simulink model "RS_O_yalmip"  (R2016b)
settings: Solver=ode1  StartTime=0.0  StopTime=T  FixedStep=1e-4  MaxStep=1e-3  RelTol=1e-6  EnableMultiTasking=on
InitFcn:
  | RS_O_script;
values from neighbouring files (symbols this model uses):
  C1 = 1e-9    (= 1e-09)    [Dati_MPC.m]
  C2 = 1e-9    (= 1e-09)    [Dati_MPC.m]
  Cext_Bp1 = Ce_Bp1*np_Bp1/ns_Bp1    (= 35750)    [Dati_MPC.m]
  Cext_Bp2 = Ce_Bp2*np_Bp2/ns_Bp2    (= 35750)    [Dati_MPC.m]
  Cext_BpM = Ce_BpM*np_BpM/ns_BpM    (= 68250)    [Dati_MPC.m]
  Cin_Bp1 = Ci_Bp1*np_Bp1/ns_Bp1    (= 16500)    [Dati_MPC.m]
  Cin_Bp2 = Ci_Bp2*np_Bp2/ns_Bp2    (= 16500)    [Dati_MPC.m]
  Cin_BpM = Ci_BpM*np_BpM/ns_BpM    (= 31500)    [Dati_MPC.m]
  Cint = 18e-3    (= 0.018)    [Dati_MPC.m]
  f = 50    [Dati_rete.m]
  ft_F = 10    [Dati_MPC.m]
  I_u = 0.1    [Dati_MPC.m]
  ki_PLL = w_t/Vd*(-w_t+sqrt(2*w_t^2-Vd^2*kp_PLL^2))    [Dati_MPC.m]
  kp_PLL = 0.9*kp_PLL_max    [Dati_MPC.m]
  MPCpar = struct    [Dati_MPC.m]    (also in Initialization.m)
  netdata = struct    [Dati_rete.m]
  P1 = 750e3    (= 750000)    [RS_O_script.m]
  P1v = 500e3    (= 500000)    [RS_O_script.m]
  P2 = 750e3    (= 750000)    [RS_O_script.m]
  P2v = 250e3    (= 250000)    [RS_O_script.m]
  P_u = 0.005    [Dati_MPC.m]
  Ppv1 = 500e3    (= 500000)    [Dati_MPC.m]
  Ppv2 = 850e3    (= 850000)    [Dati_MPC.m]
  Q1 = 350e3    (= 350000)    [RS_O_script.m]
  Q1v = 250e3    (= 250000)    [RS_O_script.m]
  Q2 = 300e3    (= 300000)    [RS_O_script.m]
  Q2v = 250e3    (= 250000)    [RS_O_script.m]
  Qbat1 = 50e3    (= 50000)    [Dati_MPC.m]
  Qbat2 = 50e3    (= 50000)    [Dati_MPC.m]
  Rext_Bp1 = Re_Bp1*ns_Bp1/np_Bp1    (= 0.0154545454545)    [Dati_MPC.m]
  Rext_Bp2 = Re_Bp2*ns_Bp2/np_Bp2    (= 0.0154545454545)    [Dati_MPC.m]
  Rext_BpM = Re_BpM*ns_BpM/np_BpM    (= 0.00809523809524)    [Dati_MPC.m]
  Rin_Bp1 = Ri_Bp1*ns_Bp1/np_Bp1    (= 0.363636363636)    [Dati_MPC.m]
  Rin_Bp2 = Ri_Bp2*ns_Bp2/np_Bp2    (= 0.363636363636)    [Dati_MPC.m]
  Rin_BpM = Ri_BpM*ns_BpM/np_BpM    (= 0.190476190476)    [Dati_MPC.m]
  SOC_10 = (Vbat1-Vbat1_min)/(Vbat1_max-Vbat1_min)    (= 0.625)    [Dati_MPC.m]
  SOC_20 = (Vbat2-Vbat2_min)/(Vbat2_max-Vbat2_min)    (= 0.625)    [Dati_MPC.m]
  SOC_M0 = (VbatM-VbatM_min)/(VbatM_max-VbatM_min)    (= 0.625)    [Dati_MPC.m]
  Srif = 1e6    (= 1000000)    [Dati_rete.m]
  t1 = 50    [RS_O_script.m]
  t2 = 110    [RS_O_script.m]
  t3 = 170    [RS_O_script.m]
  t_start_MPC = 10    [RS_O_script.m]
  tPLL = 2    [RS_O_script.m]
  Vbat1_max = 1.2*Vbat1_min    (= 480)    [Dati_MPC.m]
  Vbat1_min = 400    [Dati_MPC.m]
  Vbat2_max = 1.2*Vbat2_min    (= 480)    [Dati_MPC.m]
  Vbat2_min = 400    [Dati_MPC.m]
  VbatM_max = 1.2*VbatM_min    (= 480)    [Dati_MPC.m]
  VbatM_min = 400    [Dati_MPC.m]
  Vdc_1 = 800    [Dati_MPC.m]
  Vdc_2 = 800    [Dati_MPC.m]
  Vdc_M = 800    [Dati_MPC.m]
  Vrif_M = sqrt(2)/sqrt(3)*20e3    [Dati_MPC.m]
  Zrif = Vrif^2/Srif    (= 400)    [Dati_rete.m]
undefined symbols (not defined in the file or in its folder): Cfsc, Csc, j, L2, Lf, magnitude, Rc, Rint, Rsc
libraries: powerlib x87, powerlib_meascontrol x58, simulink x2
(part 2 of 3)

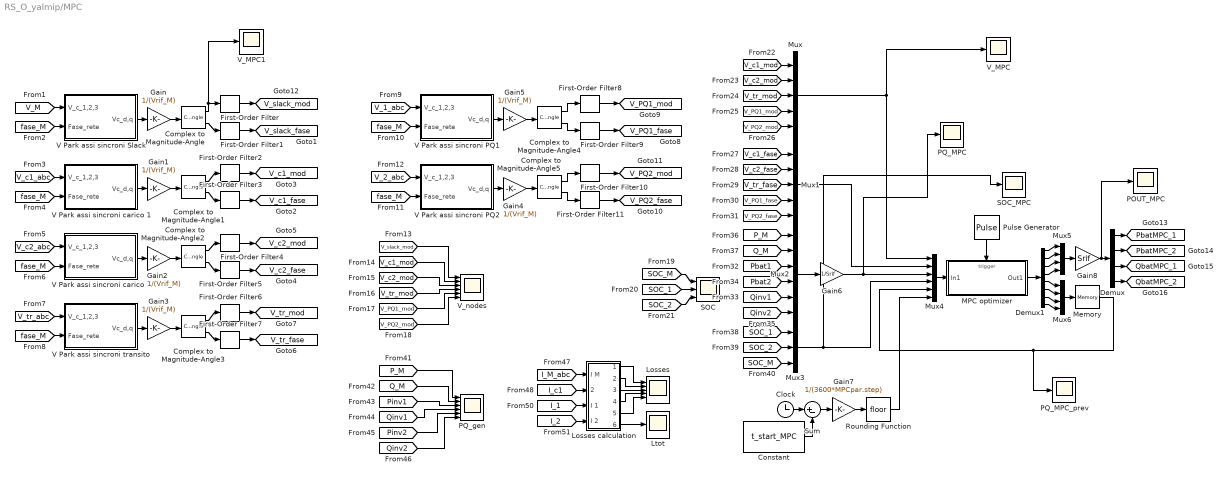
== system RS_O_yalmip/MPC ==
  Clock : Clock
  Complex to Magnitude-Angle{,1..5} (6 alike) : ComplexToMagnitudeAngle
  Constant : Constant  Value=t_start_MPC
  Demux : Demux
  Demux1 : Demux  Outputs=8
  First-Order Filter{,1..11} (12 alike) : powerlib_meascontrol/Filters/First-Order Filter  FilterType=Lowpass  Tc=1/(2*pi*ft_F)  Ts=0  Initialize=on  Vac_Init=[0, 0, 60]  Vdc_Init=0  PlotResponse=off  FreqRange="[0,  200,  1]"
  Gain{,1..5} (6 alike) : Gain  Gain=1/(Vrif_M)
  Gain6 : Gain  Gain=1/Srif
  Gain7 : Gain  Gain=1/(3600*MPCpar.step)
  Gain8 : Gain  Gain=Srif
  Losses : Scope  NumInputPorts=5
  Losses calculation : Subsystem
  Ltot : Scope
  MPC optimizer : Subsystem  TreatAsAtomicUnit=on
  Memory : Memory
  Mux : Mux  Inputs=5
  Mux1 : Mux  Inputs=5
  Mux2 : Mux  Inputs=6
  Mux3 : Mux  Inputs=3
  Mux4 : Mux  Inputs=6
  Mux5 : Mux
  Mux6 : Mux
  POUT_MPC : Scope
  PQ_MPC : Scope
  PQ_MPC_prev : Scope
  PQ_gen : Scope  NumInputPorts=6
  Pulse Generator : DiscretePulseGenerator  PulseType=Time based  Period=MPCpar.step*3600  PulseWidth=5  PhaseDelay=t_start_MPC
  Rounding Function : Rounding
  SOC : Scope  NumInputPorts=3
  SOC_MPC : Scope
  Sum : Sum  Inputs=|+-
  V Park assi sincroni PQ1 : Subsystem
  V Park assi sincroni PQ2 : Subsystem
  V Park assi sincroni Slack : Subsystem
  V Park assi sincroni carico 1 : Subsystem
  V Park assi sincroni carico 2 : Subsystem
  V Park assi sincroni transito : Subsystem
  V_MPC : Scope
  V_MPC1 : Scope
  V_nodes : Scope  NumInputPorts=6
  tag scope: PbatMPC_1=global, PbatMPC_2=global, QbatMPC_1=global, QbatMPC_2=global, V_PQ1_fase=global, V_PQ1_mod=global, V_PQ2_fase=global, V_PQ2_mod=global, V_c1_fase=global, V_c1_mod=global, V_c2_fase=global, V_c2_mod=global, V_slack_fase=global, V_slack_mod=global, V_tr_fase=global, V_tr_mod=global
  wires:
  [fase_M] -> V Park assi sincroni Slack/2(Fase_rete)
  [V_M] -> V Park assi sincroni Slack/1(V_c_1,2,3)
  [fase_M] -> V Park assi sincroni carico 1/2(Fase_rete)
  [V_c1_abc] -> V Park assi sincroni carico 1/1(V_c_1,2,3)
  [fase_M] -> V Park assi sincroni carico 2/2(Fase_rete)
  [V_c2_abc] -> V Park assi sincroni carico 2/1(V_c_1,2,3)
  [fase_M] -> V Park assi sincroni transito/2(Fase_rete)
  [V_tr_abc] -> V Park assi sincroni transito/1(V_c_1,2,3)
  [fase_M] -> V Park assi sincroni PQ1/2(Fase_rete)
  [V_1_abc] -> V Park assi sincroni PQ1/1(V_c_1,2,3)
  [fase_M] -> V Park assi sincroni PQ2/2(Fase_rete)
  [V_2_abc] -> V Park assi sincroni PQ2/1(V_c_1,2,3)
  V Park assi sincroni Slack/1(Vc_d,q) -> Gain/1
  Complex to Magnitude-Angle/1 -> V_MPC1/1, First-Order Filter/1
  Complex to Magnitude-Angle/2 -> First-Order Filter1/1
  Complex to Magnitude-Angle1/1 -> First-Order Filter2/1
  Complex to Magnitude-Angle1/2 -> First-Order Filter3/1
  V Park assi sincroni carico 1/1(Vc_d,q) -> Gain1/1
  Complex to Magnitude-Angle2/1 -> First-Order Filter4/1
  Complex to Magnitude-Angle2/2 -> First-Order Filter5/1
  V Park assi sincroni carico 2/1(Vc_d,q) -> Gain2/1
  Complex to Magnitude-Angle3/1 -> First-Order Filter6/1
  Complex to Magnitude-Angle3/2 -> First-Order Filter7/1
  V Park assi sincroni transito/1(Vc_d,q) -> Gain3/1
  Complex to Magnitude-Angle4/1 -> First-Order Filter8/1
  Complex to Magnitude-Angle4/2 -> First-Order Filter9/1
  V Park assi sincroni PQ1/1(Vc_d,q) -> Gain5/1
  Complex to Magnitude-Angle5/1 -> First-Order Filter10/1
  Complex to Magnitude-Angle5/2 -> First-Order Filter11/1
  V Park assi sincroni PQ2/1(Vc_d,q) -> Gain4/1
  [V_slack_mod] -> V_nodes/1
  [V_c1_mod] -> V_nodes/2
  [V_c2_mod] -> V_nodes/3
  [V_tr_mod] -> V_nodes/4
  [V_PQ1_mod] -> V_nodes/5
  [V_PQ2_mod] -> V_nodes/6
  Gain/1 -> Complex to Magnitude-Angle/1
  Gain1/1 -> Complex to Magnitude-Angle1/1
  Gain2/1 -> Complex to Magnitude-Angle2/1
  Gain3/1 -> Complex to Magnitude-Angle3/1
  Gain5/1 -> Complex to Magnitude-Angle4/1
  Gain4/1 -> Complex to Magnitude-Angle5/1
  [SOC_M] -> SOC/1
  [SOC_1] -> SOC/2
  [SOC_2] -> SOC/3
  First-Order Filter/1 -> [V_slack_mod]
  First-Order Filter1/1 -> [V_slack_fase]
  First-Order Filter2/1 -> [V_c1_mod]
  First-Order Filter3/1 -> [V_c1_fase]
  First-Order Filter4/1 -> [V_c2_mod]
  First-Order Filter5/1 -> [V_c2_fase]
  First-Order Filter6/1 -> [V_tr_mod]
  First-Order Filter7/1 -> [V_tr_fase]
  First-Order Filter8/1 -> [V_PQ1_mod]
  First-Order Filter9/1 -> [V_PQ1_fase]
  First-Order Filter10/1 -> [V_PQ2_mod]
  First-Order Filter11/1 -> [V_PQ2_fase]
  [V_c1_mod] -> Mux/1
  [V_c2_mod] -> Mux/2
  [V_tr_mod] -> Mux/3
  [V_PQ1_mod] -> Mux/4
  [V_PQ2_mod] -> Mux/5
  [V_c1_fase] -> Mux1/1
  [V_c2_fase] -> Mux1/2
  [V_tr_fase] -> Mux1/3
  [V_PQ1_fase] -> Mux1/4
  [V_PQ2_fase] -> Mux1/5
  [Qinv2] -> Mux2/6
  [Qinv1] -> Mux2/5
  [Pbat2] -> Mux2/4
  [Pbat1] -> Mux2/3
  [P_M] -> Mux2/1
  [Q_M] -> Mux2/2
  [SOC_1] -> Mux3/1
  [SOC_2] -> Mux3/2
  [SOC_M] -> Mux3/3
  Mux/1 -> Mux4/1, V_MPC/1
  Mux1/1 -> Mux4/2
  Mux2/1 -> Gain6/1
  Gain6/1 -> PQ_MPC/1, Mux4/3
  Mux3/1 -> SOC_MPC/1, Mux4/4
  Mux4/1 -> MPC optimizer/1(In1)
  Pulse Generator/1 -> MPC optimizer/Trigger
  Demux/1 -> [PbatMPC_1]
  Demux/2 -> [PbatMPC_2]
  Demux/4 -> [QbatMPC_2]
  Demux/3 -> [QbatMPC_1]
  Clock/1 -> Sum/1
  Constant/1 -> Sum/2
  Sum/1 -> Gain7/1
  Gain7/1 -> Rounding Function/1
  MPC optimizer/1(Out1) -> Demux1/1
  Mux5/1 -> Gain8/1
  Demux1/1 -> Mux5/1
  Demux1/2 -> Mux5/2
  Demux1/3 -> Mux5/3
  Demux1/4 -> Mux5/4
  Demux1/5 -> Mux6/1
  Demux1/6 -> Mux6/2
  Demux1/7 -> Mux6/3
  Demux1/8 -> Mux6/4
  Mux6/1 -> Memory/1
  Rounding Function/1 -> Mux4/6
  Memory/1 -> PQ_MPC_prev/1, Mux4/5
  Gain8/1 -> POUT_MPC/1, Demux/1
  [P_M] -> PQ_gen/1
  [Q_M] -> PQ_gen/2
  [Pinv1] -> PQ_gen/3
  [Qinv1] -> PQ_gen/4
  [Pinv2] -> PQ_gen/5
  [Qinv2] -> PQ_gen/6
  [I_M_abc] -> Losses calculation/1(I M)
  [I_c1] -> Losses calculation/2(I C1)
  [I_1] -> Losses calculation/3(I 1)
  [I_2] -> Losses calculation/4(I 2)
  Losses calculation/1(L12) -> Losses/1
  Losses calculation/2(L23) -> Losses/2
  Losses calculation/3(L34) -> Losses/3
  Losses calculation/4(L45) -> Losses/4
  Losses calculation/5(L46) -> Losses/5
  Losses calculation/6(Ltot) -> Ltot/1

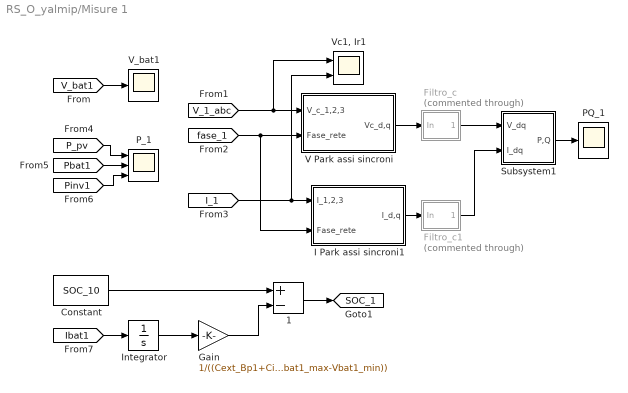
== system RS_O_yalmip/Misure 1 ==
  1 : Sum  Inputs=+-
  Constant : Constant  Value=SOC_10
  Filtro_c : Subsystem  Commented=through
  Filtro_c1 : Subsystem  Commented=through
  Gain : Gain  Gain=1/((Cext_Bp1+Cin_Bp1)*(Vbat1_max-Vbat1_min))
  I Park assi sincroni1 : Subsystem
  Integrator : Integrator
  PQ_1 : Scope
  P_1 : Scope  NumInputPorts=3
  Subsystem1 : Subsystem
  V Park assi sincroni : Subsystem
  V_bat1 : Scope
  "Vc1, Ir1" : Scope  NumInputPorts=2
  tag scope: SOC_1=global
  wires:
  I Park assi sincroni1/1(I_d,q) -> Filtro_c1/1(In)
  V Park assi sincroni/1(Vc_d,q) -> Filtro_c/1(In)
  [fase_1] -> V Park assi sincroni/2(Fase_rete), I Park assi sincroni1/2(Fase_rete)
  [I_1] -> "Vc1, Ir1"/2, I Park assi sincroni1/1(I_1,2,3)
  Subsystem1/1(P,Q) -> PQ_1/1
  [V_1_abc] -> V Park assi sincroni/1(V_c_1,2,3), "Vc1, Ir1"/1
  [P_pv] -> P_1/1
  [Pbat1] -> P_1/2
  [Pinv1] -> P_1/3
  [V_bat1] -> V_bat1/1
  [Ibat1] -> Integrator/1
  Integrator/1 -> Gain/1
  Constant/1 -> 1/1
  1/1 -> [SOC_1]
  Gain/1 -> 1/2
  Filtro_c/1(Out) -> Subsystem1/1(V_dq)
  Filtro_c1/1(Out) -> Subsystem1/2(I_dq)

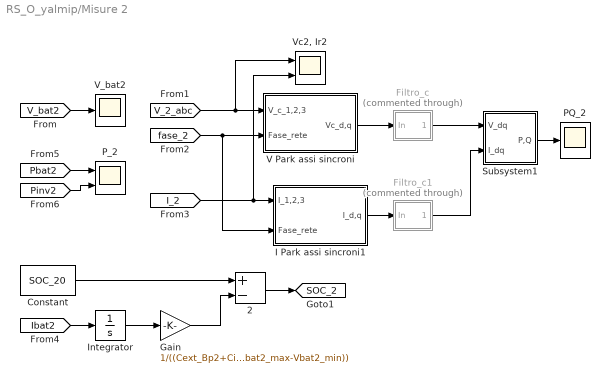
== system RS_O_yalmip/Misure 2 ==
  2 : Sum  Inputs=+-
  Constant : Constant  Value=SOC_20
  Filtro_c : Subsystem  Commented=through
  Filtro_c1 : Subsystem  Commented=through
  Gain : Gain  Gain=1/((Cext_Bp2+Cin_Bp2)*(Vbat2_max-Vbat2_min))
  I Park assi sincroni1 : Subsystem
  Integrator : Integrator
  PQ_2 : Scope
  P_2 : Scope  NumInputPorts=2
  Subsystem1 : Subsystem
  V Park assi sincroni : Subsystem
  V_bat2 : Scope
  "Vc2, Ir2" : Scope  NumInputPorts=2
  tag scope: SOC_2=global
  wires:
  [V_2_abc] -> "Vc2, Ir2"/1, V Park assi sincroni/1(V_c_1,2,3)
  Subsystem1/1(P,Q) -> PQ_2/1
  [I_2] -> I Park assi sincroni1/1(I_1,2,3), "Vc2, Ir2"/2
  [fase_2] -> I Park assi sincroni1/2(Fase_rete), V Park assi sincroni/2(Fase_rete)
  V Park assi sincroni/1(Vc_d,q) -> Filtro_c/1(In)
  I Park assi sincroni1/1(I_d,q) -> Filtro_c1/1(In)
  [V_bat2] -> V_bat2/1
  [Pinv2] -> P_2/2
  [Pbat2] -> P_2/1
  [Ibat2] -> Integrator/1
  Integrator/1 -> Gain/1
  Constant/1 -> 2/1
  2/1 -> [SOC_2]
  Gain/1 -> 2/2
  Filtro_c1/1(Out) -> Subsystem1/2(I_dq)
  Filtro_c/1(Out) -> Subsystem1/1(V_dq)

== system RS_O_yalmip/Misure Carichi ==
  First-Order Filter{,1..3} (4 alike) : powerlib_meascontrol/Filters/First-Order Filter  FilterType=Lowpass  Tc=1/(2*pi*ft_F)  Ts=0  Initialize=on  Vac_Init=[0, 0, 60]  Vdc_Init=0  PlotResponse=off  FreqRange="[0,  200,  1]"
  PQ_c1 : Scope  NumInputPorts=2
  PQ_c2 : Scope  NumInputPorts=2
  P_c1,2 : Scope  NumInputPorts=4
  "Power (3ph, Instantaneous)" : powerlib_meascontrol/Measurements/Power (3ph, Instantaneous)
  "Power (3ph, Instantaneous)1" : powerlib_meascontrol/Measurements/Power (3ph, Instantaneous)
  V,I_c1 : Scope  NumInputPorts=2
  V,I_c2 : Scope  NumInputPorts=2
  tag scope: Pc1=global, Pc2=global, Qc1=global, Qc2=global
  wires:
  [I_c1] -> "Power (3ph, Instantaneous)"/2, V,I_c1/2
  [V_c1_abc] -> "Power (3ph, Instantaneous)"/1, V,I_c1/1
  "Power (3ph, Instantaneous)"/2 -> First-Order Filter1/1
  "Power (3ph, Instantaneous)1"/2 -> First-Order Filter3/1
  "Power (3ph, Instantaneous)1"/1 -> First-Order Filter2/1
  [I_c2] -> "Power (3ph, Instantaneous)1"/2, V,I_c2/2
  [V_c2_abc] -> "Power (3ph, Instantaneous)1"/1, V,I_c2/1
  "Power (3ph, Instantaneous)"/1 -> First-Order Filter/1
  First-Order Filter/1 -> [Pc1], P_c1,2/1, PQ_c1/1
  First-Order Filter1/1 -> P_c1,2/2, [Qc1], PQ_c1/2
  First-Order Filter2/1 -> P_c1,2/3, [Pc2], PQ_c2/1
  First-Order Filter3/1 -> P_c1,2/4, [Qc2], PQ_c2/2

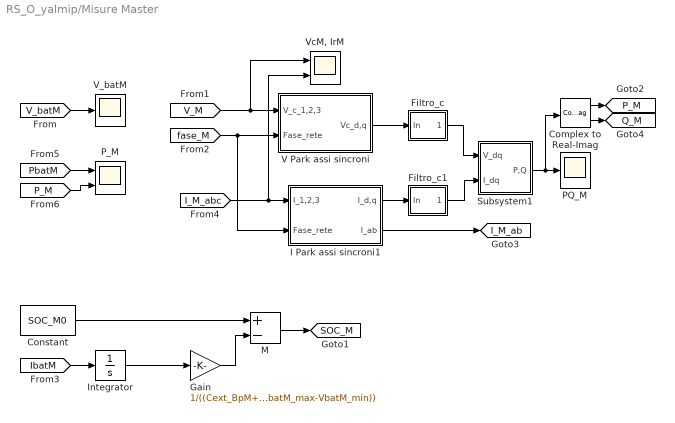
== system RS_O_yalmip/Misure Master ==
  Complex to Real-Imag : ComplexToRealImag
  Constant : Constant  Value=SOC_M0
  Filtro_c : Subsystem
  Filtro_c1 : Subsystem
  Gain : Gain  Gain=1/((Cext_BpM+Cin_BpM)*(VbatM_max-VbatM_min))
  I Park assi sincroni1 : Subsystem
  Integrator : Integrator
  M : Sum  Inputs=+-
  PQ_M : Scope
  P_M : Scope  NumInputPorts=2
  Subsystem1 : Subsystem
  V Park assi sincroni : Subsystem
  V_batM : Scope
  "VcM, IrM" : Scope  NumInputPorts=2
  tag scope: I_M_ab=global, P_M=global, Q_M=global, SOC_M=global
  wires:
  Subsystem1/1(P,Q) -> PQ_M/1, Complex to Real-Imag/1
  [I_M_abc] -> I Park assi sincroni1/1(I_1,2,3), "VcM, IrM"/2
  [fase_M] -> I Park assi sincroni1/2(Fase_rete), V Park assi sincroni/2(Fase_rete)
  [V_M] -> "VcM, IrM"/1, V Park assi sincroni/1(V_c_1,2,3)
  I Park assi sincroni1/2(I_ab) -> [I_M_ab]
  V Park assi sincroni/1(Vc_d,q) -> Filtro_c/1(In)
  I Park assi sincroni1/1(I_d,q) -> Filtro_c1/1(In)
  [P_M] -> P_M/2
  [PbatM] -> P_M/1
  [V_batM] -> V_batM/1
  [IbatM] -> Integrator/1
  Integrator/1 -> Gain/1
  Constant/1 -> M/1
  M/1 -> [SOC_M]
  Gain/1 -> M/2
  Filtro_c/1(Out) -> Subsystem1/1(V_dq)
  Filtro_c1/1(Out) -> Subsystem1/2(I_dq)
  Complex to Real-Imag/2 -> [Q_M]
  Complex to Real-Imag/1 -> [P_M]

== system RS_O_yalmip/Misure transito ==
  Subsystem2 : Subsystem
  Three-Phase Series RLC Load2 : powerlib/Elements/Three-Phase Series RLC Load  LConnTagsString=A|B|C  Configuration=Y (floating)  NominalVoltage=20e3  Vabc=[1e3 1e3 1e3]  Vabcp=[1e3 1e3 1e3]  NominalFrequency=50  UnbalancedPower=off  ActivePower=0.1  InductivePower=0  CapacitivePower=0  Pabc=[10e3 9e3 11e3]  QLabc=[100 90 110]  QCabc=[100 90 110]  Pabcp=[10e3 9e3 11e3]  QLabcp=[100 90 110]  QCabcp=[100 90 110]  Measurements=None  LoadType=constant PQ
  Three-Phase V-I Measurement2 : powerlib/Measurements/Three-Phase V-I Measurement  VoltageMeasurement=phase-to-phase  SetLabelV=off  LabelV=Vabc  Vpu=off  VpuLL=off  CurrentMeasurement=no  SetLabelI=off  LabelI=Iabc  Ipu=off  Pbase=100e6  Vbase=500e3  OutputType=Complex  PhasorSimulation=off  PSBequivalent=0
  A : PMIOPort  Port=1  Side=Left
  B : PMIOPort  Port=2  Side=Left
  C : PMIOPort  Port=3  Side=Left
  tag scope: V_tr_abc=global
  wires:
  Three-Phase V-I Measurement2/1 -> Subsystem2/1(V_c)
  Subsystem2/1(V_f) -> [V_tr_abc]
  connections:
  Three-Phase V-I Measurement2/RConn1 -- Three-Phase Series RLC Load2/LConn1
  Three-Phase Series RLC Load2/LConn3 -- Three-Phase V-I Measurement2/RConn3
  Three-Phase Series RLC Load2/LConn2 -- Three-Phase V-I Measurement2/RConn2
  Three-Phase V-I Measurement2/LConn2 -- B/RConn1
  Three-Phase V-I Measurement2/LConn3 -- C/RConn1
  Three-Phase V-I Measurement2/LConn1 -- A/RConn1

== system RS_O_yalmip/Carico1/PLL ==
  V_a,b : Inport
  Add1 : Sum
  Complex to Real-Imag : ComplexToRealImag  Output=Imag
  Complex to Real-Imag1 : ComplexToRealImag  Output=Real
  Constant2 : Constant  Value=50
  Filtro_c : Subsystem
  Gain2 : Gain  Gain=-j
  Gain3 : Gain  Gain=2*pi
  Integrator : Integrator  WrapState=on
  Math Function1 : Math  SaturateOnIntegerOverflow=on
  PI_fase : Subsystem
  Product1 : Product
  Vs : Outport
  Fase : Outport  Port=2
  wires:
  Complex to Real-Imag1/1 -> Vs/1
  Add1/1 -> Integrator/1
  Filtro_c/1(Out) -> Complex to Real-Imag1/1
  V_a,b/1 -> Product1/1
  Integrator/1 -> Gain2/1, Fase/1
  Complex to Real-Imag/1 -> PI_fase/1(dI)
  Product1/1 -> Complex to Real-Imag/1, Filtro_c/1(In)
  Constant2/1 -> Gain3/1
  Gain3/1 -> Add1/2
  Gain2/1 -> Math Function1/1
  Math Function1/1 -> Product1/2
  PI_fase/1(dw) -> Add1/1

== system RS_O_yalmip/Carico1/Park su assi fissi ==
  V_1,2,3 : Inport
  Add : Sum  Inputs=+++
  Constant : Constant  Value=exp(j*2*pi/3)
  Constant1 : Constant  Value=exp(j*4*pi/3)
  Demux : Demux  Outputs=3
  Gain : Gain  Gain=2/3
  Product : Product
  Product1 : Product
  V_s : Outport
  wires:
  Demux/2 -> Product/1
  Product/1 -> Add/2
  Product1/1 -> Add/3
  Constant/1 -> Product/2
  Constant1/1 -> Product1/2
  Add/1 -> Gain/1
  Demux/3 -> Product1/1
  Gain/1 -> V_s/1
  V_1,2,3/1 -> Demux/1
  Demux/1 -> Add/1

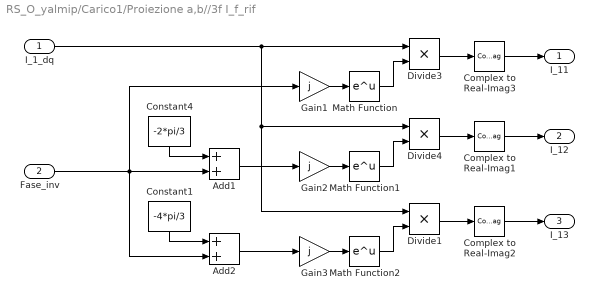
== system RS_O_yalmip/Carico1/Proiezione a,b//3f I_f_rif ==
  I_1_dq : Inport
  Fase_inv : Inport  Port=2
  Add1 : Sum
  Add2 : Sum
  Complex to Real-Imag1 : ComplexToRealImag  Output=Real
  Complex to Real-Imag2 : ComplexToRealImag  Output=Real
  Complex to Real-Imag3 : ComplexToRealImag  Output=Real
  Constant1 : Constant  Value=-4*pi/3
  Constant4 : Constant  Value=-2*pi/3
  Divide1 : Product  Inputs=**
  Divide3 : Product  Inputs=**
  Divide4 : Product  Inputs=**
  Gain1 : Gain  Gain=j
  Gain2 : Gain  Gain=j
  Gain3 : Gain  Gain=j
  Math Function : Math  SaturateOnIntegerOverflow=on
  Math Function1 : Math  SaturateOnIntegerOverflow=on
  Math Function2 : Math  SaturateOnIntegerOverflow=on
  I_11 : Outport
  I_12 : Outport  Port=2
  I_13 : Outport  Port=3
  wires:
  Constant1/1 -> Add2/1
  Constant4/1 -> Add1/1
  Fase_inv/1 -> Add1/2, Add2/2, Gain1/1
  Add2/1 -> Gain3/1
  Add1/1 -> Gain2/1
  Math Function2/1 -> Divide1/2
  Gain3/1 -> Math Function2/1
  I_1_dq/1 -> Divide3/1, Divide4/1, Divide1/1
  Math Function1/1 -> Divide4/2
  Gain2/1 -> Math Function1/1
  Math Function/1 -> Divide3/2
  Gain1/1 -> Math Function/1
  Complex to Real-Imag2/1 -> I_13/1
  Complex to Real-Imag1/1 -> I_12/1
  Complex to Real-Imag3/1 -> I_11/1
  Divide1/1 -> Complex to Real-Imag2/1
  Divide4/1 -> Complex to Real-Imag1/1
  Divide3/1 -> Complex to Real-Imag3/1

== system RS_O_yalmip/Carico1/Ritardo_PLL1 ==
  P : Inport
  Divide6 : Product  Inputs=**
  Step : Step  Time=tPLL  SampleTime=0
  g : Outport
  wires:
  P/1 -> Divide6/1
  Divide6/1 -> g/1
  Step/1 -> Divide6/2

== system RS_O_yalmip/Carico1/Ritardo_PLL2 ==
  P : Inport
  Divide6 : Product  Inputs=**
  Step : Step  Time=tPLL  SampleTime=0
  g : Outport
  wires:
  Step/1 -> Divide6/2
  Divide6/1 -> g/1
  P/1 -> Divide6/1

== system RS_O_yalmip/Carico1/Ritardo_PLL7 ==
  P : Inport
  Divide6 : Product  Inputs=**
  Step : Step  Time=tPLL  SampleTime=0
  g : Outport
  wires:
  Step/1 -> Divide6/2
  Divide6/1 -> g/1
  P/1 -> Divide6/1

== system RS_O_yalmip/Carico1/Subsystem ==
  P : Inport
  Q : Inport  Port=2
  V : Inport  Port=3
  Divide5 : Product  Inputs=*/
  Divide6 : Product  Inputs=*/
  First-Order Filter : powerlib_meascontrol/Filters/First-Order Filter  FilterType=Lowpass  Tc=1/(2*pi*ft_F)  Ts=0  Initialize=on  Vac_Init=[0, 0, 60]  Vdc_Init=0  PlotResponse=off  FreqRange="[0,  200,  1]"
  First-Order Filter1 : powerlib_meascontrol/Filters/First-Order Filter  FilterType=Lowpass  Tc=1/(2*pi*ft_F)  Ts=0  Initialize=on  Vac_Init=[0, 0, 60]  Vdc_Init=0  PlotResponse=off  FreqRange="[0,  200,  1]"
  Gain : Gain  Gain=2/3
  Gain2 : Gain  Gain=2/3
  Gain3 : Gain  Gain=-1
  Real-Imag to Complex : RealImagToComplex
  Saturation : Saturate  UpperLimit=inf  LowerLimit=1e-6
  I_dq : Outport
  wires:
  Gain3/1 -> Divide6/2
  V/1 -> Saturation/1
  Real-Imag to Complex/1 -> I_dq/1
  P/1 -> Gain/1
  Gain2/1 -> Divide6/1
  Gain/1 -> Divide5/1
  Q/1 -> Gain2/1
  Saturation/1 -> Divide5/2, Gain3/1
  Divide5/1 -> First-Order Filter/1
  Divide6/1 -> First-Order Filter1/1
  First-Order Filter/1 -> Real-Imag to Complex/1
  First-Order Filter1/1 -> Real-Imag to Complex/2

== system RS_O_yalmip/Carico1/Subsystem1 ==
  V_c : Inport
  Add : Sum  Inputs=+-
  Add1 : Sum  Inputs=+-
  Add2 : Sum  Inputs=+-
  Demux : Demux  Outputs=3
  Gain : Gain  Gain=1/3
  Gain1 : Gain  Gain=1/3
  Gain2 : Gain  Gain=1/3
  Mux2 : Mux  Inputs=3
  V_f : Outport
  wires:
  Mux2/1 -> V_f/1
  Demux/1 -> Gain/1
  Gain/1 -> Add1/2, Add/1
  Demux/2 -> Gain1/1
  Gain2/1 -> Add/2, Add2/1
  Gain1/1 -> Add2/2, Add1/1
  Add/1 -> Mux2/1
  Add1/1 -> Mux2/2
  Add2/1 -> Mux2/3
  V_c/1 -> Demux/1
  Demux/3 -> Gain2/1

== system RS_O_yalmip/Carico2/PLL ==
  V_a,b : Inport
  Add1 : Sum
  Complex to Real-Imag : ComplexToRealImag  Output=Imag
  Complex to Real-Imag1 : ComplexToRealImag  Output=Real
  Constant2 : Constant  Value=50
  Filtro_c : Subsystem
  Gain2 : Gain  Gain=-j
  Gain3 : Gain  Gain=2*pi
  Integrator : Integrator  WrapState=on
  Math Function1 : Math  SaturateOnIntegerOverflow=on
  PI_fase : Subsystem
  Product1 : Product
  Vs : Outport
  Fase : Outport  Port=2
  wires:
  Complex to Real-Imag1/1 -> Vs/1
  Add1/1 -> Integrator/1
  Filtro_c/1(Out) -> Complex to Real-Imag1/1
  V_a,b/1 -> Product1/1
  Integrator/1 -> Gain2/1, Fase/1
  Complex to Real-Imag/1 -> PI_fase/1(dI)
  Product1/1 -> Complex to Real-Imag/1, Filtro_c/1(In)
  Constant2/1 -> Gain3/1
  Gain3/1 -> Add1/2
  Gain2/1 -> Math Function1/1
  Math Function1/1 -> Product1/2
  PI_fase/1(dw) -> Add1/1

== system RS_O_yalmip/Carico2/Park su assi fissi ==
  V_1,2,3 : Inport
  Add : Sum  Inputs=+++
  Constant : Constant  Value=exp(j*2*pi/3)
  Constant1 : Constant  Value=exp(j*4*pi/3)
  Demux : Demux  Outputs=3
  Gain : Gain  Gain=2/3
  Product : Product
  Product1 : Product
  V_s : Outport
  wires:
  Demux/2 -> Product/1
  Product/1 -> Add/2
  Product1/1 -> Add/3
  Constant/1 -> Product/2
  Constant1/1 -> Product1/2
  Add/1 -> Gain/1
  Demux/3 -> Product1/1
  Gain/1 -> V_s/1
  V_1,2,3/1 -> Demux/1
  Demux/1 -> Add/1

== system RS_O_yalmip/Carico2/Proiezione a,b//3f I_f_rif ==
  I_1_dq : Inport
  Fase_inv : Inport  Port=2
  Add1 : Sum
  Add2 : Sum
  Complex to Real-Imag1 : ComplexToRealImag  Output=Real
  Complex to Real-Imag2 : ComplexToRealImag  Output=Real
  Complex to Real-Imag3 : ComplexToRealImag  Output=Real
  Constant1 : Constant  Value=-4*pi/3
  Constant4 : Constant  Value=-2*pi/3
  Divide1 : Product  Inputs=**
  Divide3 : Product  Inputs=**
  Divide4 : Product  Inputs=**
  Gain1 : Gain  Gain=j
  Gain2 : Gain  Gain=j
  Gain3 : Gain  Gain=j
  Math Function : Math  SaturateOnIntegerOverflow=on
  Math Function1 : Math  SaturateOnIntegerOverflow=on
  Math Function2 : Math  SaturateOnIntegerOverflow=on
  I_11 : Outport
  I_12 : Outport  Port=2
  I_13 : Outport  Port=3
  wires:
  Constant1/1 -> Add2/1
  Constant4/1 -> Add1/1
  Fase_inv/1 -> Add1/2, Add2/2, Gain1/1
  Add2/1 -> Gain3/1
  Add1/1 -> Gain2/1
  Math Function2/1 -> Divide1/2
  Gain3/1 -> Math Function2/1
  I_1_dq/1 -> Divide3/1, Divide4/1, Divide1/1
  Math Function1/1 -> Divide4/2
  Gain2/1 -> Math Function1/1
  Math Function/1 -> Divide3/2
  Gain1/1 -> Math Function/1
  Complex to Real-Imag2/1 -> I_13/1
  Complex to Real-Imag1/1 -> I_12/1
  Complex to Real-Imag3/1 -> I_11/1
  Divide1/1 -> Complex to Real-Imag2/1
  Divide4/1 -> Complex to Real-Imag1/1
  Divide3/1 -> Complex to Real-Imag3/1

== system RS_O_yalmip/Carico2/Ritardo_PLL1 ==
  P : Inport
  Divide6 : Product  Inputs=**
  Step : Step  Time=tPLL  SampleTime=0
  g : Outport
  wires:
  P/1 -> Divide6/1
  Divide6/1 -> g/1
  Step/1 -> Divide6/2

== system RS_O_yalmip/Carico2/Ritardo_PLL2 ==
  P : Inport
  Divide6 : Product  Inputs=**
  Step : Step  Time=tPLL  SampleTime=0
  g : Outport
  wires:
  Step/1 -> Divide6/2
  Divide6/1 -> g/1
  P/1 -> Divide6/1

== system RS_O_yalmip/Carico2/Ritardo_PLL7 ==
  P : Inport
  Divide6 : Product  Inputs=**
  Step : Step  Time=tPLL  SampleTime=0
  g : Outport
  wires:
  Step/1 -> Divide6/2
  Divide6/1 -> g/1
  P/1 -> Divide6/1

== system RS_O_yalmip/Carico2/Subsystem ==
  P : Inport
  Q : Inport  Port=2
  V : Inport  Port=3
  Divide5 : Product  Inputs=*/
  Divide6 : Product  Inputs=*/
  First-Order Filter : powerlib_meascontrol/Filters/First-Order Filter  FilterType=Lowpass  Tc=1/(2*pi*ft_F)  Ts=0  Initialize=on  Vac_Init=[0, 0, 60]  Vdc_Init=0  PlotResponse=off  FreqRange="[0,  200,  1]"
  First-Order Filter1 : powerlib_meascontrol/Filters/First-Order Filter  FilterType=Lowpass  Tc=1/(2*pi*ft_F)  Ts=0  Initialize=on  Vac_Init=[0, 0, 60]  Vdc_Init=0  PlotResponse=off  FreqRange="[0,  200,  1]"
  Gain : Gain  Gain=2/3
  Gain2 : Gain  Gain=2/3
  Gain3 : Gain  Gain=-1
  Real-Imag to Complex : RealImagToComplex
  Saturation : Saturate  UpperLimit=inf  LowerLimit=1e-6
  I_dq : Outport
  wires:
  Gain3/1 -> Divide6/2
  V/1 -> Saturation/1
  Real-Imag to Complex/1 -> I_dq/1
  P/1 -> Gain/1
  Gain2/1 -> Divide6/1
  Gain/1 -> Divide5/1
  Q/1 -> Gain2/1
  Saturation/1 -> Divide5/2, Gain3/1
  Divide5/1 -> First-Order Filter/1
  Divide6/1 -> First-Order Filter1/1
  First-Order Filter/1 -> Real-Imag to Complex/1
  First-Order Filter1/1 -> Real-Imag to Complex/2

== system RS_O_yalmip/Carico2/Subsystem1 ==
  V_c : Inport
  Add : Sum  Inputs=+-
  Add1 : Sum  Inputs=+-
  Add2 : Sum  Inputs=+-
  Demux : Demux  Outputs=3
  Gain : Gain  Gain=1/3
  Gain1 : Gain  Gain=1/3
  Gain2 : Gain  Gain=1/3
  Mux2 : Mux  Inputs=3
  V_f : Outport
  wires:
  Mux2/1 -> V_f/1
  Demux/1 -> Gain/1
  Gain/1 -> Add1/2, Add/1
  Demux/2 -> Gain1/1
  Gain2/1 -> Add/2, Add2/1
  Gain1/1 -> Add2/2, Add1/1
  Add/1 -> Mux2/1
  Add1/1 -> Mux2/2
  Add2/1 -> Mux2/3
  V_c/1 -> Demux/1
  Demux/3 -> Gain2/1

== system RS_O_yalmip/Controllo 1/PLL ==
  V_a,b : Inport
  Add1 : Sum
  Complex to Real-Imag : ComplexToRealImag  Output=Imag
  Complex to Real-Imag1 : ComplexToRealImag  Output=Real
  Constant2 : Constant  Value=50
  Filtro_c : Subsystem
  Gain2 : Gain  Gain=-j
  Gain3 : Gain  Gain=2*pi
  Integrator : Integrator  WrapState=on
  Math Function1 : Math  SaturateOnIntegerOverflow=on
  PI_fase : Subsystem
  Product1 : Product
  Vs : Outport
  Fase : Outport  Port=2
  wires:
  Complex to Real-Imag1/1 -> Vs/1
  Add1/1 -> Integrator/1
  Filtro_c/1(Out) -> Complex to Real-Imag1/1
  V_a,b/1 -> Product1/1
  Integrator/1 -> Gain2/1, Fase/1
  Complex to Real-Imag/1 -> PI_fase/1(dI)
  Product1/1 -> Complex to Real-Imag/1, Filtro_c/1(In)
  Constant2/1 -> Gain3/1
  Gain3/1 -> Add1/2
  Gain2/1 -> Math Function1/1
  Math Function1/1 -> Product1/2
  PI_fase/1(dw) -> Add1/1

== system RS_O_yalmip/Controllo 1/Park su assi fissi ==
  V_1,2,3 : Inport
  Add : Sum  Inputs=+++
  Constant : Constant  Value=exp(j*2*pi/3)
  Constant1 : Constant  Value=exp(j*4*pi/3)
  Demux : Demux  Outputs=3
  Gain : Gain  Gain=2/3
  Product : Product
  Product1 : Product
  V_s : Outport
  wires:
  Demux/2 -> Product/1
  Product/1 -> Add/2
  Product1/1 -> Add/3
  Constant/1 -> Product/2
  Constant1/1 -> Product1/2
  Add/1 -> Gain/1
  Demux/3 -> Product1/1
  Gain/1 -> V_s/1
  V_1,2,3/1 -> Demux/1
  Demux/1 -> Add/1

== system RS_O_yalmip/Controllo 1/Proiezione a,b//3f I_f_rif ==
  I_1_dq : Inport
  Fase_inv : Inport  Port=2
  Add1 : Sum
  Add2 : Sum
  Complex to Real-Imag1 : ComplexToRealImag  Output=Real
  Complex to Real-Imag2 : ComplexToRealImag  Output=Real
  Complex to Real-Imag3 : ComplexToRealImag  Output=Real
  Constant1 : Constant  Value=-4*pi/3
  Constant4 : Constant  Value=-2*pi/3
  Divide1 : Product  Inputs=**
  Divide3 : Product  Inputs=**
  Divide4 : Product  Inputs=**
  Gain1 : Gain  Gain=j
  Gain2 : Gain  Gain=j
  Gain3 : Gain  Gain=j
  Math Function : Math  SaturateOnIntegerOverflow=on
  Math Function1 : Math  SaturateOnIntegerOverflow=on
  Math Function2 : Math  SaturateOnIntegerOverflow=on
  I_11 : Outport
  I_12 : Outport  Port=2
  I_13 : Outport  Port=3
  wires:
  Constant1/1 -> Add2/1
  Constant4/1 -> Add1/1
  Fase_inv/1 -> Add1/2, Add2/2, Gain1/1
  Add2/1 -> Gain3/1
  Add1/1 -> Gain2/1
  Math Function2/1 -> Divide1/2
  Gain3/1 -> Math Function2/1
  I_1_dq/1 -> Divide3/1, Divide4/1, Divide1/1
  Math Function1/1 -> Divide4/2
  Gain2/1 -> Math Function1/1
  Math Function/1 -> Divide3/2
  Gain1/1 -> Math Function/1
  Complex to Real-Imag2/1 -> I_13/1
  Complex to Real-Imag1/1 -> I_12/1
  Complex to Real-Imag3/1 -> I_11/1
  Divide1/1 -> Complex to Real-Imag2/1
  Divide4/1 -> Complex to Real-Imag1/1
  Divide3/1 -> Complex to Real-Imag3/1

== system RS_O_yalmip/Controllo 1/Ritardo_PLL1 ==
  P : Inport
  Divide6 : Product  Inputs=**
  Step : Step  Time=tPLL  SampleTime=0
  g : Outport
  wires:
  P/1 -> Divide6/1
  Divide6/1 -> g/1
  Step/1 -> Divide6/2

== system RS_O_yalmip/Controllo 1/Ritardo_PLL2 ==
  P : Inport
  Divide6 : Product  Inputs=**
  Step : Step  Time=tPLL  SampleTime=0
  g : Outport
  wires:
  Step/1 -> Divide6/2
  Divide6/1 -> g/1
  P/1 -> Divide6/1

== system RS_O_yalmip/Controllo 1/Ritardo_PLL3 ==
  P : Inport
  Divide6 : Product  Inputs=**
  Step : Step  Time=tPLL  SampleTime=0
  g : Outport
  wires:
  P/1 -> Divide6/1
  Divide6/1 -> g/1
  Step/1 -> Divide6/2

== system RS_O_yalmip/Controllo 1/Ritardo_PLL7 ==
  P : Inport
  Divide6 : Product  Inputs=**
  Step : Step  Time=tPLL  SampleTime=0
  g : Outport
  wires:
  Step/1 -> Divide6/2
  Divide6/1 -> g/1
  P/1 -> Divide6/1

== system RS_O_yalmip/Controllo 1/Subsystem ==
  P : Inport
  Q : Inport  Port=2
  V : Inport  Port=3
  Divide5 : Product  Inputs=*/
  Divide6 : Product  Inputs=*/
  First-Order Filter : powerlib_meascontrol/Filters/First-Order Filter  Commented=through  FilterType=Lowpass  Tc=1/(2*pi*ft_F)  Ts=0  Initialize=on  Vac_Init=[0, 0, 60]  Vdc_Init=0  PlotResponse=off  FreqRange="[0,  200,  1]"
  First-Order Filter1 : powerlib_meascontrol/Filters/First-Order Filter  Commented=through  FilterType=Lowpass  Tc=1/(2*pi*ft_F)  Ts=0  Initialize=on  Vac_Init=[0, 0, 60]  Vdc_Init=0  PlotResponse=off  FreqRange="[0,  200,  1]"
  Gain : Gain  Gain=2/3
  Gain2 : Gain  Gain=2/3
  Gain3 : Gain  Gain=-1
  Real-Imag to Complex : RealImagToComplex
  Saturation : Saturate  UpperLimit=inf  LowerLimit=1e-6
  I_dq : Outport
  wires:
  Gain3/1 -> Divide6/2
  V/1 -> Saturation/1
  Real-Imag to Complex/1 -> I_dq/1
  P/1 -> Gain/1
  Gain2/1 -> Divide6/1
  Gain/1 -> Divide5/1
  Q/1 -> Gain2/1
  Saturation/1 -> Divide5/2, Gain3/1
  Divide5/1 -> First-Order Filter/1
  Divide6/1 -> First-Order Filter1/1
  First-Order Filter/1 -> Real-Imag to Complex/1
  First-Order Filter1/1 -> Real-Imag to Complex/2

== system RS_O_yalmip/Controllo 2/PLL ==
  V_a,b : Inport
  Add1 : Sum
  Complex to Real-Imag : ComplexToRealImag  Output=Imag
  Complex to Real-Imag1 : ComplexToRealImag  Output=Real
  Constant2 : Constant  Value=50
  Filtro_c : Subsystem
  Gain2 : Gain  Gain=-j
  Gain3 : Gain  Gain=2*pi
  Integrator : Integrator  WrapState=on
  Math Function1 : Math  SaturateOnIntegerOverflow=on
  PI_fase : Subsystem
  Product1 : Product
  Vs : Outport
  Fase : Outport  Port=2
  wires:
  Complex to Real-Imag1/1 -> Vs/1
  Add1/1 -> Integrator/1
  Filtro_c/1(Out) -> Complex to Real-Imag1/1
  V_a,b/1 -> Product1/1
  Integrator/1 -> Gain2/1, Fase/1
  Complex to Real-Imag/1 -> PI_fase/1(dI)
  Product1/1 -> Complex to Real-Imag/1, Filtro_c/1(In)
  Constant2/1 -> Gain3/1
  Gain3/1 -> Add1/2
  Gain2/1 -> Math Function1/1
  Math Function1/1 -> Product1/2
  PI_fase/1(dw) -> Add1/1

== system RS_O_yalmip/Controllo 2/Park su assi fissi ==
  V_1,2,3 : Inport
  Add : Sum  Inputs=+++
  Constant : Constant  Value=exp(j*2*pi/3)
  Constant1 : Constant  Value=exp(j*4*pi/3)
  Demux : Demux  Outputs=3
  Gain : Gain  Gain=2/3
  Product : Product
  Product1 : Product
  V_s : Outport
  wires:
  Demux/2 -> Product/1
  Product/1 -> Add/2
  Product1/1 -> Add/3
  Constant/1 -> Product/2
  Constant1/1 -> Product1/2
  Add/1 -> Gain/1
  Demux/3 -> Product1/1
  Gain/1 -> V_s/1
  V_1,2,3/1 -> Demux/1
  Demux/1 -> Add/1

== system RS_O_yalmip/Controllo 2/Proiezione a,b//3f I_f_rif ==
  I_1_dq : Inport
  Fase_inv : Inport  Port=2
  Add1 : Sum
  Add2 : Sum
  Complex to Real-Imag1 : ComplexToRealImag  Output=Real
  Complex to Real-Imag2 : ComplexToRealImag  Output=Real
  Complex to Real-Imag3 : ComplexToRealImag  Output=Real
  Constant1 : Constant  Value=-4*pi/3
  Constant4 : Constant  Value=-2*pi/3
  Divide1 : Product  Inputs=**
  Divide3 : Product  Inputs=**
  Divide4 : Product  Inputs=**
  Gain1 : Gain  Gain=j
  Gain2 : Gain  Gain=j
  Gain3 : Gain  Gain=j
  Math Function : Math  SaturateOnIntegerOverflow=on
  Math Function1 : Math  SaturateOnIntegerOverflow=on
  Math Function2 : Math  SaturateOnIntegerOverflow=on
  I_11 : Outport
  I_12 : Outport  Port=2
  I_13 : Outport  Port=3
  wires:
  Constant1/1 -> Add2/1
  Constant4/1 -> Add1/1
  Fase_inv/1 -> Add1/2, Add2/2, Gain1/1
  Add2/1 -> Gain3/1
  Add1/1 -> Gain2/1
  Math Function2/1 -> Divide1/2
  Gain3/1 -> Math Function2/1
  I_1_dq/1 -> Divide3/1, Divide4/1, Divide1/1
  Math Function1/1 -> Divide4/2
  Gain2/1 -> Math Function1/1
  Math Function/1 -> Divide3/2
  Gain1/1 -> Math Function/1
  Complex to Real-Imag2/1 -> I_13/1
  Complex to Real-Imag1/1 -> I_12/1
  Complex to Real-Imag3/1 -> I_11/1
  Divide1/1 -> Complex to Real-Imag2/1
  Divide4/1 -> Complex to Real-Imag1/1
  Divide3/1 -> Complex to Real-Imag3/1

== system RS_O_yalmip/Controllo 2/Ritardo_PLL1 ==
  P : Inport
  Divide6 : Product  Inputs=**
  Step : Step  Time=tPLL  SampleTime=0
  g : Outport
  wires:
  P/1 -> Divide6/1
  Divide6/1 -> g/1
  Step/1 -> Divide6/2

== system RS_O_yalmip/Controllo 2/Ritardo_PLL2 ==
  P : Inport
  Divide6 : Product  Inputs=**
  Step : Step  Time=tPLL  SampleTime=0
  g : Outport
  wires:
  Step/1 -> Divide6/2
  Divide6/1 -> g/1
  P/1 -> Divide6/1

== system RS_O_yalmip/Controllo 2/Ritardo_PLL3 ==
  P : Inport
  Divide6 : Product  Inputs=**
  Step : Step  Time=tPLL  SampleTime=0
  g : Outport
  wires:
  P/1 -> Divide6/1
  Divide6/1 -> g/1
  Step/1 -> Divide6/2

== system RS_O_yalmip/Controllo 2/Ritardo_PLL7 ==
  P : Inport
  Divide6 : Product  Inputs=**
  Step : Step  Time=tPLL  SampleTime=0
  g : Outport
  wires:
  Step/1 -> Divide6/2
  Divide6/1 -> g/1
  P/1 -> Divide6/1

== system RS_O_yalmip/Controllo 2/Subsystem ==
  P : Inport
  Q : Inport  Port=2
  V : Inport  Port=3
  Divide5 : Product  Inputs=*/
  Divide6 : Product  Inputs=*/
  First-Order Filter : powerlib_meascontrol/Filters/First-Order Filter  Commented=through  FilterType=Lowpass  Tc=1/(2*pi*ft_F)  Ts=0  Initialize=on  Vac_Init=[0, 0, 60]  Vdc_Init=0  PlotResponse=off  FreqRange="[0,  200,  1]"
  First-Order Filter1 : powerlib_meascontrol/Filters/First-Order Filter  Commented=through  FilterType=Lowpass  Tc=1/(2*pi*ft_F)  Ts=0  Initialize=on  Vac_Init=[0, 0, 60]  Vdc_Init=0  PlotResponse=off  FreqRange="[0,  200,  1]"
  Gain : Gain  Gain=2/3
  Gain2 : Gain  Gain=2/3
  Gain3 : Gain  Gain=-1
  Real-Imag to Complex : RealImagToComplex
  Saturation : Saturate  UpperLimit=inf  LowerLimit=1e-6
  I_dq : Outport
  wires:
  Gain3/1 -> Divide6/2
  V/1 -> Saturation/1
  Real-Imag to Complex/1 -> I_dq/1
  P/1 -> Gain/1
  Gain2/1 -> Divide6/1
  Gain/1 -> Divide5/1
  Q/1 -> Gain2/1
  Saturation/1 -> Divide5/2, Gain3/1
  Divide5/1 -> First-Order Filter/1
  Divide6/1 -> First-Order Filter1/1
  First-Order Filter/1 -> Real-Imag to Complex/1
  First-Order Filter1/1 -> Real-Imag to Complex/2

== system RS_O_yalmip/Controllo Master/Media complessa ==
  w : Inport
  fase : Inport  Port=2
  I_a,b : Inport  Port=3
  Complex to Real-Imag : ComplexToRealImag
  Divide3 : Product  Inputs=**
  Filtro_c1 : Subsystem
  Gain : Gain  Gain=1/(2*pi)
  Gain1 : Gain  Gain=-j
  Math Function : Math  SaturateOnIntegerOverflow=on
  Mean (Variable Frequency) : powerlib_meascontrol/Measurements/Mean (Variable Frequency)  Finit=50  Fmin=45  Vinit=0  Ts=0
  Mean (Variable Frequency)1 : powerlib_meascontrol/Measurements/Mean (Variable Frequency)  Finit=50  Fmin=45  Vinit=0  Ts=0
  Real-Imag to Complex : RealImagToComplex
  I_dc_d,q : Outport
  wires:
  I_a,b/1 -> Complex to Real-Imag/1
  Complex to Real-Imag/1 -> Mean (Variable Frequency)/2
  Complex to Real-Imag/2 -> Mean (Variable Frequency)1/2
  Mean (Variable Frequency)/1 -> Real-Imag to Complex/1
  Mean (Variable Frequency)1/1 -> Real-Imag to Complex/2
  w/1 -> Gain/1
  Gain/1 -> Mean (Variable Frequency)1/1, Mean (Variable Frequency)/1
  Gain1/1 -> Math Function/1
  Math Function/1 -> Divide3/2
  Divide3/1 -> I_dc_d,q/1
  fase/1 -> Gain1/1
  Real-Imag to Complex/1 -> Filtro_c1/1(In)
  Filtro_c1/1(Out) -> Divide3/1

== system RS_O_yalmip/Controllo Master/PI Complesso ==
  In1 : Inport
  Complex to Real-Imag : ComplexToRealImag
  Gain1 : Gain  Gain=-1
  PID Controller : simulink/Continuous/PID Controller  Controller=PI  TimeDomain=Continuous-time  SampleTime=-1  IntegratorMethod=Forward Euler  FilterMethod=Forward Euler  Form=Parallel  UseFilter=on  ControllerParametersSource=internal  P=P_u  I=I_u  D=0  N=100  InitialConditionSource=internal  InitialConditionForIntegrator=0  InitialConditionForFilter=0  ExternalReset=none  LimitOutput=off  UpperSaturationLimit=inf  LowerSaturationLimit=-inf  LinearizeAsGain=on  AntiWindupMode=none  Kb=1  TrackingMode=off  Kt=1  PParamMin=[]  PParamMax=[]  IParamMin=[]  IParamMax=[]  DParamMin=[]  DParamMax=[]  NParamMin=[]  NParamMax=[]  KbParamMin=[]  KbParamMax=[]  KtParamMin=[]  KtParamMax=[]  POutMin=[]  POutMax=[]  IOutMin=[]  IOutMax=[]  DOutMin=[]  DOutMax=[]  NOutMin=[]  NOutMax=[]  KbOutMin=[]  KbOutMax=[]  KtOutMin=[]  KtOutMax=[]  IntegratorOutMin=[]  IntegratorOutMax=[]  FilterOutMin=[]  FilterOutMax=[]  SumOutMin=[]  SumOutMax=[]  SumI1OutMin=[]  SumI1OutMax=[]  SumI2OutMin=[]  SumI2OutMax=[]  SumI3OutMin=[]  SumI3OutMax=[]  SumDOutMin=[]  SumDOutMax=[]  SaturationOutMin=[]  SaturationOutMax=[]  IntegratorContinuousStateAttributes=''  IntegratorStateMustResolveToSignalObject=off  IntegratorRTWStateStorageClass=Auto  FilterContinuousStateAttributes=''  FilterStateMustResolveToSignalObject=off  FilterRTWStateStorageClass=Auto  DifferentiatorICPrevScaledInput=0  DifferentiatorOutMin=[]  DifferentiatorOutMax=[]
  PID Controller1 : simulink/Continuous/PID Controller  Controller=PI  TimeDomain=Continuous-time  SampleTime=-1  IntegratorMethod=Forward Euler  FilterMethod=Forward Euler  Form=Parallel  UseFilter=on  ControllerParametersSource=internal  P=P_u  I=I_u  D=0  N=100  InitialConditionSource=internal  InitialConditionForIntegrator=0  InitialConditionForFilter=0  ExternalReset=none  LimitOutput=off  UpperSaturationLimit=inf  LowerSaturationLimit=-inf  LinearizeAsGain=on  AntiWindupMode=none  Kb=1  TrackingMode=off  Kt=1  PParamMin=[]  PParamMax=[]  IParamMin=[]  IParamMax=[]  DParamMin=[]  DParamMax=[]  NParamMin=[]  NParamMax=[]  KbParamMin=[]  KbParamMax=[]  KtParamMin=[]  KtParamMax=[]  POutMin=[]  POutMax=[]  IOutMin=[]  IOutMax=[]  DOutMin=[]  DOutMax=[]  NOutMin=[]  NOutMax=[]  KbOutMin=[]  KbOutMax=[]  KtOutMin=[]  KtOutMax=[]  IntegratorOutMin=[]  IntegratorOutMax=[]  FilterOutMin=[]  FilterOutMax=[]  SumOutMin=[]  SumOutMax=[]  SumI1OutMin=[]  SumI1OutMax=[]  SumI2OutMin=[]  SumI2OutMax=[]  SumI3OutMin=[]  SumI3OutMax=[]  SumDOutMin=[]  SumDOutMax=[]  SaturationOutMin=[]  SaturationOutMax=[]  IntegratorContinuousStateAttributes=''  IntegratorStateMustResolveToSignalObject=off  IntegratorRTWStateStorageClass=Auto  FilterContinuousStateAttributes=''  FilterStateMustResolveToSignalObject=off  FilterRTWStateStorageClass=Auto  DifferentiatorICPrevScaledInput=0  DifferentiatorOutMin=[]  DifferentiatorOutMax=[]
  Real-Imag to Complex : RealImagToComplex
  Out1 : Outport
  wires:
  In1/1 -> Gain1/1
  Gain1/1 -> Complex to Real-Imag/1
  Complex to Real-Imag/1 -> PID Controller/1
  Complex to Real-Imag/2 -> PID Controller1/1
  PID Controller/1 -> Real-Imag to Complex/1
  PID Controller1/1 -> Real-Imag to Complex/2
  Real-Imag to Complex/1 -> Out1/1

== system RS_O_yalmip/Controllo Master/Proiezione a,b//3f I_f_rif ==
  V_M_dq : Inport
  Fase_inv : Inport  Port=2
  Add1 : Sum
  Add2 : Sum
  Complex to Real-Imag1 : ComplexToRealImag  Output=Real
  Complex to Real-Imag2 : ComplexToRealImag  Output=Real
  Complex to Real-Imag3 : ComplexToRealImag  Output=Real
  Constant1 : Constant  Value=-4*pi/3
  Constant4 : Constant  Value=-2*pi/3
  Divide1 : Product  Inputs=**
  Divide3 : Product  Inputs=**
  Divide4 : Product  Inputs=**
  Gain1 : Gain  Gain=j
  Gain2 : Gain  Gain=j
  Gain3 : Gain  Gain=j
  Math Function : Math  SaturateOnIntegerOverflow=on
  Math Function1 : Math  SaturateOnIntegerOverflow=on
  Math Function2 : Math  SaturateOnIntegerOverflow=on
  V_M1 : Outport
  V_M2 : Outport  Port=2
  V_M3 : Outport  Port=3
  wires:
  Divide3/1 -> Complex to Real-Imag3/1
  Divide4/1 -> Complex to Real-Imag1/1
  Divide1/1 -> Complex to Real-Imag2/1
  Complex to Real-Imag3/1 -> V_M1/1
  Complex to Real-Imag1/1 -> V_M2/1
  Complex to Real-Imag2/1 -> V_M3/1
  Gain1/1 -> Math Function/1
  Math Function/1 -> Divide3/2
  Gain2/1 -> Math Function1/1
  Math Function1/1 -> Divide4/2
  V_M_dq/1 -> Divide1/1, Divide4/1, Divide3/1
  Gain3/1 -> Math Function2/1
  Math Function2/1 -> Divide1/2
  Add1/1 -> Gain2/1
  Add2/1 -> Gain3/1
  Fase_inv/1 -> Gain1/1, Add2/2, Add1/2
  Constant4/1 -> Add1/1
  Constant1/1 -> Add2/1

== system RS_O_yalmip/DC PV/Ritardo_PLL2 ==
  P : Inport
  Divide6 : Product  Inputs=**
  Step : Step  Time=tPLL  SampleTime=0
  g : Outport
  wires:
  Step/1 -> Divide6/2
  Divide6/1 -> g/1
  P/1 -> Divide6/1

== system RS_O_yalmip/Inverter ID 1/Subsystem2 ==
  V_c : Inport
  Add : Sum  Inputs=+-
  Add1 : Sum  Inputs=+-
  Add2 : Sum  Inputs=+-
  Demux : Demux  Outputs=3
  Gain : Gain  Gain=1/3
  Gain1 : Gain  Gain=1/3
  Gain2 : Gain  Gain=1/3
  Mux2 : Mux  Inputs=3
  V_f : Outport
  wires:
  Mux2/1 -> V_f/1
  Demux/1 -> Gain/1
  Gain/1 -> Add1/2, Add/1
  Demux/2 -> Gain1/1
  Gain2/1 -> Add/2, Add2/1
  Gain1/1 -> Add2/2, Add1/1
  Add/1 -> Mux2/1
  Add1/1 -> Mux2/2
  Add2/1 -> Mux2/3
  V_c/1 -> Demux/1
  Demux/3 -> Gain2/1

== system RS_O_yalmip/Inverter ID 2/Subsystem2 ==
  V_c : Inport
  Add : Sum  Inputs=+-
  Add1 : Sum  Inputs=+-
  Add2 : Sum  Inputs=+-
  Demux : Demux  Outputs=3
  Gain : Gain  Gain=1/3
  Gain1 : Gain  Gain=1/3
  Gain2 : Gain  Gain=1/3
  Mux2 : Mux  Inputs=3
  V_f : Outport
  wires:
  Demux/3 -> Gain2/1
  V_c/1 -> Demux/1
  Add2/1 -> Mux2/3
  Add1/1 -> Mux2/2
  Add/1 -> Mux2/1
  Gain1/1 -> Add1/1, Add2/2
  Gain2/1 -> Add2/1, Add/2
  Demux/2 -> Gain1/1
  Gain/1 -> Add/1, Add1/2
  Demux/1 -> Gain/1
  Mux2/1 -> V_f/1

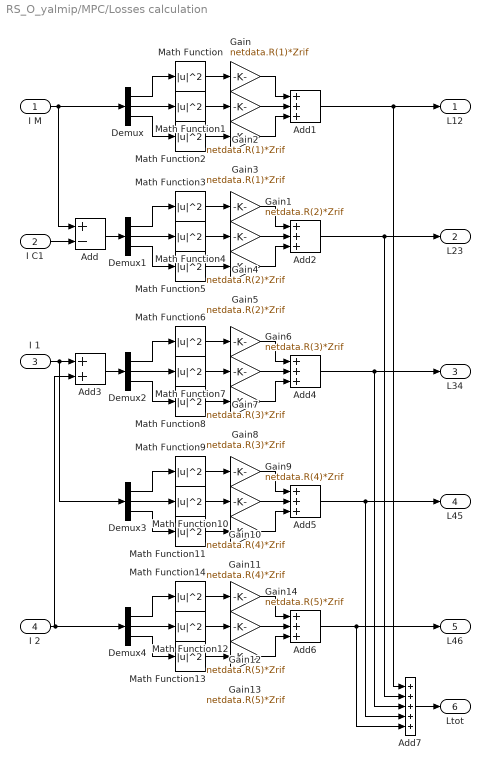
== system RS_O_yalmip/MPC/Losses calculation ==
  I M : Inport
  I C1 : Inport  Port=2
  I 1 : Inport  Port=3
  I 2 : Inport  Port=4
  Add : Sum  Inputs=+-
  Add{1..2,4..6} (5 alike) : Sum  Inputs=+++
  Add3 : Sum
  Add7 : Sum  Inputs=+++++
  Demux{,1..4} (5 alike) : Demux  Outputs=3
  Gain : Gain  Gain=netdata.R(1)*Zrif
  Gain1 : Gain  Gain=netdata.R(2)*Zrif
  Gain10 : Gain  Gain=netdata.R(4)*Zrif
  Gain11 : Gain  Gain=netdata.R(4)*Zrif
  Gain12 : Gain  Gain=netdata.R(5)*Zrif
  Gain13 : Gain  Gain=netdata.R(5)*Zrif
  Gain14 : Gain  Gain=netdata.R(5)*Zrif
  Gain2 : Gain  Gain=netdata.R(1)*Zrif
  Gain3 : Gain  Gain=netdata.R(1)*Zrif
  Gain4 : Gain  Gain=netdata.R(2)*Zrif
  Gain5 : Gain  Gain=netdata.R(2)*Zrif
  Gain6 : Gain  Gain=netdata.R(3)*Zrif
  Gain7 : Gain  Gain=netdata.R(3)*Zrif
  Gain8 : Gain  Gain=netdata.R(3)*Zrif
  Gain9 : Gain  Gain=netdata.R(4)*Zrif
  Math Function{,1..14} (15 alike) : Math  Operator=magnitude^2  SaturateOnIntegerOverflow=on
  L12 : Outport
  L23 : Outport  Port=2
  L34 : Outport  Port=3
  L45 : Outport  Port=4
  L46 : Outport  Port=5
  Ltot : Outport  Port=6
  wires:
  Math Function/1 -> Gain/1
  I C1/1 -> Add/2
  I M/1 -> Add/1, Demux/1
  Demux/1 -> Math Function/1
  Math Function1/1 -> Gain2/1
  Demux/2 -> Math Function1/1
  Math Function2/1 -> Gain3/1
  Demux/3 -> Math Function2/1
  Gain/1 -> Add1/1
  Gain2/1 -> Add1/2
  Gain3/1 -> Add1/3
  Add1/1 -> Add7/1, L12/1
  Math Function3/1 -> Gain1/1
  Demux1/1 -> Math Function3/1
  Math Function4/1 -> Gain4/1
  Demux1/2 -> Math Function4/1
  Math Function5/1 -> Gain5/1
  Demux1/3 -> Math Function5/1
  Gain1/1 -> Add2/1
  Gain4/1 -> Add2/2
  Gain5/1 -> Add2/3
  Add/1 -> Demux1/1
  Add2/1 -> Add7/2, L23/1
  Math Function6/1 -> Gain6/1
  Demux2/1 -> Math Function6/1
  Math Function7/1 -> Gain7/1
  Demux2/2 -> Math Function7/1
  Math Function8/1 -> Gain8/1
  Demux2/3 -> Math Function8/1
  Gain6/1 -> Add4/1
  Gain7/1 -> Add4/2
  Gain8/1 -> Add4/3
  Add3/1 -> Demux2/1
  Add4/1 -> Add7/3, L34/1
  I 2/1 -> Add3/2, Demux4/1
  Math Function9/1 -> Gain9/1
  I 1/1 -> Demux3/1, Add3/1
  Demux3/1 -> Math Function9/1
  Math Function10/1 -> Gain10/1
  Demux3/2 -> Math Function10/1
  Math Function11/1 -> Gain11/1
  Demux3/3 -> Math Function11/1
  Gain9/1 -> Add5/1
  Gain10/1 -> Add5/2
  Gain11/1 -> Add5/3
  Add5/1 -> Add7/4, L45/1
  Math Function14/1 -> Gain14/1
  Demux4/1 -> Math Function14/1
  Math Function12/1 -> Gain12/1
  Demux4/2 -> Math Function12/1
  Math Function13/1 -> Gain13/1
  Demux4/3 -> Math Function13/1
  Gain14/1 -> Add6/1
  Gain12/1 -> Add6/2
  Gain13/1 -> Add6/3
  Add6/1 -> Add7/5, L46/1
  Add7/1 -> Ltot/1

== system RS_O_yalmip/MPC/MPC optimizer ==
  In1 : Inport
  Trigger : TriggerPort  VariantControl=Variant
  Interpreted MATLAB Function : MATLABFcn  MATLABFcn=MPC_opt  OutputDimensions=8
  Out1 : Outport
  wires:
  Interpreted MATLAB Function/1 -> Out1/1
  In1/1 -> Interpreted MATLAB Function/1

== system RS_O_yalmip/MPC/V Park assi sincroni PQ1 ==
  V_c_1,2,3 : Inport
  Fase_rete : Inport  Port=2
  Add : Sum  Inputs=+++
  Constant : Constant  Value=exp(j*2*pi/3)
  Constant1 : Constant  Value=exp(j*4*pi/3)
  Demux : Demux  Outputs=3
  Gain : Gain  Gain=2/3
  Gain1 : Gain  Gain=-j
  Math Function : Math  SaturateOnIntegerOverflow=on
  Product : Product
  Product1 : Product
  Product2 : Product
  Vc_d,q : Outport
  wires:
  Fase_rete/1 -> Gain1/1
  Product2/1 -> Vc_d,q/1
  Gain1/1 -> Math Function/1
  Math Function/1 -> Product2/2
  Product/1 -> Add/2
  Product1/1 -> Add/3
  Constant/1 -> Product/2
  Constant1/1 -> Product1/2
  Add/1 -> Gain/1
  V_c_1,2,3/1 -> Demux/1
  Demux/1 -> Add/1
  Demux/2 -> Product/1
  Demux/3 -> Product1/1
  Gain/1 -> Product2/1

== system RS_O_yalmip/MPC/V Park assi sincroni PQ2 ==
  V_c_1,2,3 : Inport
  Fase_rete : Inport  Port=2
  Add : Sum  Inputs=+++
  Constant : Constant  Value=exp(j*2*pi/3)
  Constant1 : Constant  Value=exp(j*4*pi/3)
  Demux : Demux  Outputs=3
  Gain : Gain  Gain=2/3
  Gain1 : Gain  Gain=-j
  Math Function : Math  SaturateOnIntegerOverflow=on
  Product : Product
  Product1 : Product
  Product2 : Product
  Vc_d,q : Outport
  wires:
  Gain/1 -> Product2/1
  Demux/3 -> Product1/1
  Demux/2 -> Product/1
  Demux/1 -> Add/1
  V_c_1,2,3/1 -> Demux/1
  Add/1 -> Gain/1
  Constant1/1 -> Product1/2
  Constant/1 -> Product/2
  Product1/1 -> Add/3
  Product/1 -> Add/2
  Math Function/1 -> Product2/2
  Gain1/1 -> Math Function/1
  Product2/1 -> Vc_d,q/1
  Fase_rete/1 -> Gain1/1

== system RS_O_yalmip/MPC/V Park assi sincroni Slack ==
  V_c_1,2,3 : Inport
  Fase_rete : Inport  Port=2
  Add : Sum  Inputs=+++
  Constant : Constant  Value=exp(j*2*pi/3)
  Constant1 : Constant  Value=exp(j*4*pi/3)
  Demux : Demux  Outputs=3
  Gain : Gain  Gain=2/3
  Gain1 : Gain  Gain=-j
  Math Function : Math  SaturateOnIntegerOverflow=on
  Product : Product
  Product1 : Product
  Product2 : Product
  Vc_d,q : Outport
  wires:
  Gain/1 -> Product2/1
  Demux/3 -> Product1/1
  Demux/2 -> Product/1
  Demux/1 -> Add/1
  V_c_1,2,3/1 -> Demux/1
  Add/1 -> Gain/1
  Constant1/1 -> Product1/2
  Constant/1 -> Product/2
  Product1/1 -> Add/3
  Product/1 -> Add/2
  Math Function/1 -> Product2/2
  Gain1/1 -> Math Function/1
  Product2/1 -> Vc_d,q/1
  Fase_rete/1 -> Gain1/1

== system RS_O_yalmip/MPC/V Park assi sincroni carico 1 ==
  V_c_1,2,3 : Inport
  Fase_rete : Inport  Port=2
  Add : Sum  Inputs=+++
  Constant : Constant  Value=exp(j*2*pi/3)
  Constant1 : Constant  Value=exp(j*4*pi/3)
  Demux : Demux  Outputs=3
  Gain : Gain  Gain=2/3
  Gain1 : Gain  Gain=-j
  Math Function : Math  SaturateOnIntegerOverflow=on
  Product : Product
  Product1 : Product
  Product2 : Product
  Vc_d,q : Outport
  wires:
  Fase_rete/1 -> Gain1/1
  Product2/1 -> Vc_d,q/1
  Gain1/1 -> Math Function/1
  Math Function/1 -> Product2/2
  Product/1 -> Add/2
  Product1/1 -> Add/3
  Constant/1 -> Product/2
  Constant1/1 -> Product1/2
  Add/1 -> Gain/1
  V_c_1,2,3/1 -> Demux/1
  Demux/1 -> Add/1
  Demux/2 -> Product/1
  Demux/3 -> Product1/1
  Gain/1 -> Product2/1

== system RS_O_yalmip/MPC/V Park assi sincroni carico 2 ==
  V_c_1,2,3 : Inport
  Fase_rete : Inport  Port=2
  Add : Sum  Inputs=+++
  Constant : Constant  Value=exp(j*2*pi/3)
  Constant1 : Constant  Value=exp(j*4*pi/3)
  Demux : Demux  Outputs=3
  Gain : Gain  Gain=2/3
  Gain1 : Gain  Gain=-j
  Math Function : Math  SaturateOnIntegerOverflow=on
  Product : Product
  Product1 : Product
  Product2 : Product
  Vc_d,q : Outport
  wires:
  Fase_rete/1 -> Gain1/1
  Product2/1 -> Vc_d,q/1
  Gain1/1 -> Math Function/1
  Math Function/1 -> Product2/2
  Product/1 -> Add/2
  Product1/1 -> Add/3
  Constant/1 -> Product/2
  Constant1/1 -> Product1/2
  Add/1 -> Gain/1
  V_c_1,2,3/1 -> Demux/1
  Demux/1 -> Add/1
  Demux/2 -> Product/1
  Demux/3 -> Product1/1
  Gain/1 -> Product2/1

== system RS_O_yalmip/MPC/V Park assi sincroni transito ==
  V_c_1,2,3 : Inport
  Fase_rete : Inport  Port=2
  Add : Sum  Inputs=+++
  Constant : Constant  Value=exp(j*2*pi/3)
  Constant1 : Constant  Value=exp(j*4*pi/3)
  Demux : Demux  Outputs=3
  Gain : Gain  Gain=2/3
  Gain1 : Gain  Gain=-j
  Math Function : Math  SaturateOnIntegerOverflow=on
  Product : Product
  Product1 : Product
  Product2 : Product
  Vc_d,q : Outport
  wires:
  Gain/1 -> Product2/1
  Demux/3 -> Product1/1
  Demux/2 -> Product/1
  Demux/1 -> Add/1
  V_c_1,2,3/1 -> Demux/1
  Add/1 -> Gain/1
  Constant1/1 -> Product1/2
  Constant/1 -> Product/2
  Product1/1 -> Add/3
  Product/1 -> Add/2
  Math Function/1 -> Product2/2
  Gain1/1 -> Math Function/1
  Product2/1 -> Vc_d,q/1
  Fase_rete/1 -> Gain1/1
